simulink model "Switch1"  (Simulink 8.0)
settings: Solver=ode45  StartTime=0.0  StopTime=10.0  RelTol=1e-3
libraries: powerlib_extras x1
settings Model: Creator=Faradars  LastModifiedBy=Faradars

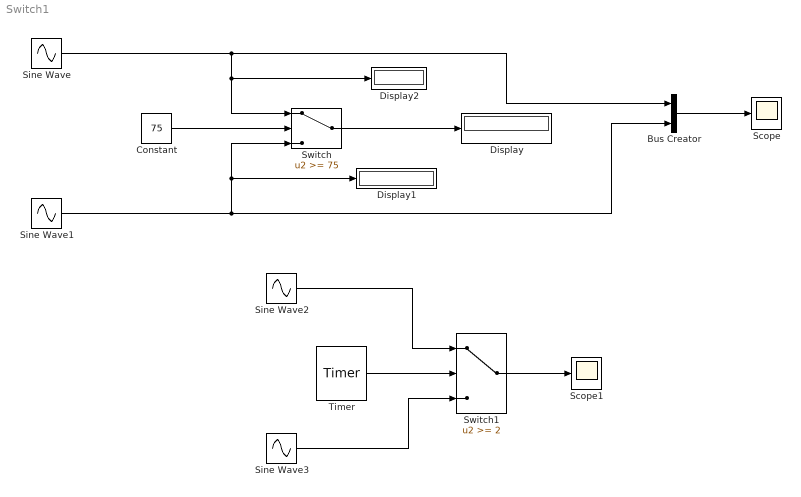
== system Switch1 ==
  Bus Creator : BusCreator  Inputs=2
  Constant : Constant  Value=75
  Display : Display
  Display1 : Display
  Display2 : Display
  Scope : Scope
  Scope1 : Scope
  Sine Wave : Sin  Bias=75  SampleTime=0
  Sine Wave1 : Sin  Bias=75  Phase=-pi  SampleTime=0
  Sine Wave2 : Sin  Bias=75  SampleTime=0
  Sine Wave3 : Sin  Bias=75  Phase=-pi  SampleTime=0
  Switch : Switch  Threshold=75
  Switch1 : Switch  Threshold=2
  Timer : powerlib_extras/Control  Blocks/Timer  t="[ 0  4  10]"  e="[1  2  3]"
  wires:
  Constant/1 -> Switch/2
  Switch/1 -> Display/1
  Sine Wave/1 -> Bus Creator/1, Switch/1, Display2/1
  Sine Wave1/1 -> Display1/1, Switch/3, Bus Creator/2
  Bus Creator/1 -> Scope/1
  Sine Wave2/1 -> Switch1/1
  Sine Wave3/1 -> Switch1/3
  Timer/1 -> Switch1/2
  Switch1/1 -> Scope1/1
